simulink model "reaction_pendulum"  (R2021b)
settings: Solver=FixedStepDiscrete  StartTime=0.0  StopTime=20  FixedStep=h  RelTol=1e-3  EnableMultiTasking=on
PreLoadFcn:
  | warning('off','MATLAB:dispatcher:InexactMatch');
InitFcn:
  | hwinit
undefined symbols (not defined in the file or in its folder): estimate_A, estimate_C, estimate_D
libraries: slident x2, dspsrcs4 x1
settings Model: SimulationMode=external  ExtModeTrigDuration=100000  Creator=user  LastModifiedBy=nstienen
settings SolverCC: AlgebraicLoopSolver=TrustRegion
settings DataIOCC: SaveFormat=Array  SignalLoggingSaveFormat=ModelDataLogs  SaveOutput=off  SignalLogging=off  DSMLogging=off  SaveTime=off  ReturnWorkspaceOutputs=off
settings OptimizationCC: ExpressionDepthLimit=2147483647  LifeSpan=inf
settings DebuggingCC: UnderspecifiedInitializationDetection=Classic  MergeDetectMultiDrivingBlocksExec=none  SolverPrmCheckMsg=warning  FcnCallInpInsideContextMsg=warning  StateNameClashWarn=warning  SFUnexpectedBacktrackingDiag=warning  SFNoUnconditionalDefaultTransitionDiag=warning  SFExecutionAtInitializationDiag=none  SFMachineParentedDataDiag=warning  ArithmeticOperatorsInVariantConditions=warning
settings HardwareCC: ProdBitPerPointer=32  ProdBitPerSizeT=32  ProdBitPerPtrDiffT=32  ProdLargestAtomicFloat=None  ProdIntDivRoundTo=Undefined  ProdEndianess=Unspecified  ProdWordSize=32  ProdHWDeviceType=32-bit Generic
settings ModelReferenceCC: PropagateSignalLabelsOutOfModel=off
settings SFSimCC: SimUseLocalCustomCode=off  CustomCodeUndefinedFunction=UseInterfaceOnly
settings RTWCC: Description=rpend RTDAC/USB2 (Visual C/C++)  SystemTargetFile=rtcon_rpend_usb2.tlc  TemplateMakefile=rtcon_rpend_vc_usb2_x64.tmf  RTWUseLocalCustomCode=off
settings CodeAppCC: StateflowObjectComments=on
settings STFCustomTargetCC: ModelReferenceCompliant=off  CombineOutputUpdateFcns=on  MatFileLogging=on  GRTInterface=off  SystemTargetFile=rtcon_rpend_usb2.tlc
settings GRTTargetCC: TargetLangStandard=C89/C90 (ANSI)  ModelReferenceCompliant=off  ParMdlRefBuildCompliant=off  CompOptLevelCompliant=off  ConcurrentExecutionCompliant=off  CPPClassGenCompliant=off  UseToolchainInfoCompliant=off  ExtMode=on  ExtModeMexFile=rtcon_ext_comm
settings ConfigComp: CovMetricSettings=dw  CovSaveCumulativeToWorkspaceVar=on  CovSaveSingleToWorkspaceVar=on  CovExternalEMLEnable=off  CovSFcnEnable=off

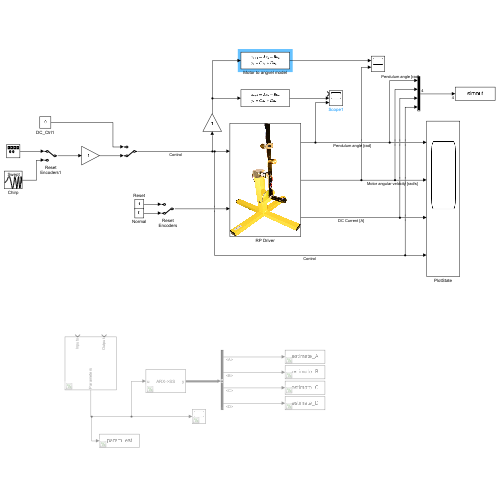
[thumbnail: Simulink's stored preview of the top-level diagram]
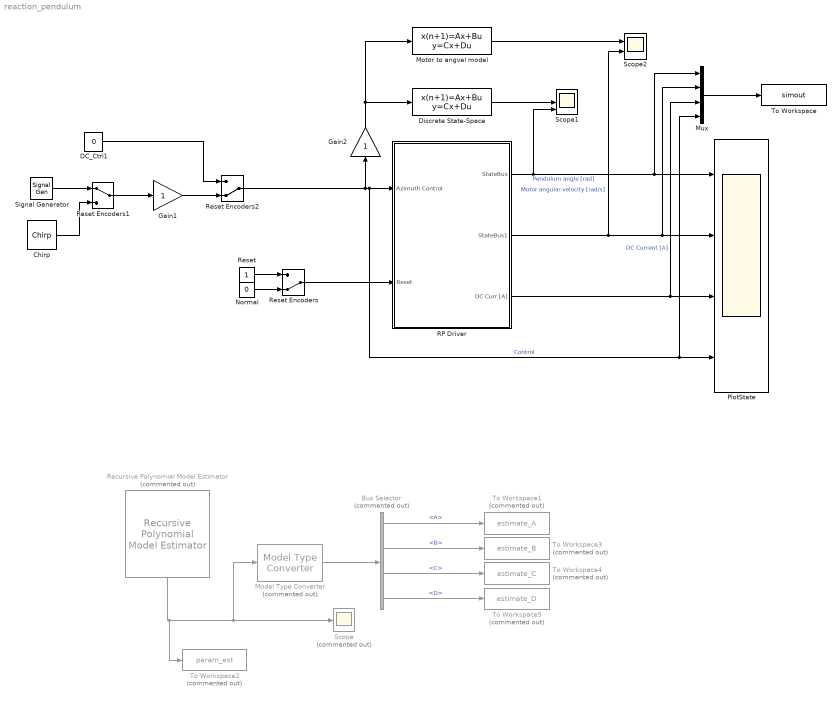
== system reaction_pendulum ==
  Bus Selector : BusSelector  Commented=on  OutputSignals=A,B,C,D
  Chirp : dspsrcs4/Chirp  sweep=Swept cosine  mode=Unidirectional  f0=0.1  f1=0.8  t1=30  Tsweep=30  phase=0  Ts=0.05  spf=1  datatype=Double  OutputFrames=off
  DC_Ctrl1 : Constant  Value=0
  Discrete State-Space : DiscreteStateSpace  A=estimate_A  B=estimate_B.'  C=estimate_C  D=estimate_D  SampleTime=-1
  Gain1 : Gain
  Gain2 : Gain
  Model Type Converter : slident/Estimators/Model Type Converter  Commented=on  InputModelType=ARX
      settings: SourceProductBaseCode=ID
  Motor to angvel model : DiscreteStateSpace  A=0.9683  B=19.81  D=0  SampleTime=-1
  Mux : Mux
  Normal : Constant  Value=0
  PlotState : Scope  NumInputPorts=4
  RP Driver : Subsystem
      mask Display: image(imread('rwp.JPG'))
  Recursive Polynomial Model Estimator : slident/Estimators/Recursive Polynomial Model Estimator  Commented=on  ModelStructure=ARX  InitialEstimateSource=None  A0=3  B0=1  C0=1  D0=1  F0=2  nk=1  P0=1e4  InitialInputs=0  InitialOutputs=0  History=Infinite  WindowLength=200  EstimationMethod=Kalman Filter  AdaptationParameter=1  HasTimeVaryingAdaptationParameter=off  NormalizationBias=eps  OutputError=off  OutputP=off  AddEnablePort=off  InputProcessing=Sample-based  Ts=-1
      settings: SourceProductBaseCode=ID
  Reset : Constant
  Reset Encoders : ManualSwitch  CurrentSetting=0
  Reset Encoders1 : ManualSwitch
  Reset Encoders2 : ManualSwitch  CurrentSetting=0
  Scope : Scope  Commented=on
  Scope1 : Scope  NumInputPorts=3
  Scope2 : Scope  NumInputPorts=2
  Signal Generator : SignalGenerator  Frequency=1/2
  To Workspace : ToWorkspace  VariableName=simout  SaveFormat=Structure With Time  SampleTime=-1
      settings: Save2DSignal=2-D array (concatenate along first dimension)
  To Workspace1 : ToWorkspace  Commented=on  VariableName=estimate_A  SampleTime=-1
      settings: MaxDataPoints=1
  To Workspace2 : ToWorkspace  Commented=on  VariableName=param_est  SaveFormat=Structure With Time  SampleTime=-1
  To Workspace3 : ToWorkspace  Commented=on  VariableName=estimate_B  SampleTime=-1
      settings: MaxDataPoints=1
  To Workspace4 : ToWorkspace  Commented=on  VariableName=estimate_C  SampleTime=-1
      settings: MaxDataPoints=1
  To Workspace5 : ToWorkspace  Commented=on  VariableName=estimate_D  SampleTime=-1
      settings: MaxDataPoints=1
  wires:
  Normal/1 -> Reset Encoders/2
  Reset/1 -> Reset Encoders/1
  Reset Encoders/1 -> RP Driver/2(Reset)
  RP Driver/3(DC Curr [A]) -> Mux/3, PlotState/3  "DC Current [A]"
  Reset Encoders2/1 -> Gain2/1, Mux/4, PlotState/4, RP Driver/1(Azimuth Control)  "Control"
  DC_Ctrl1/1 -> Reset Encoders2/1
  RP Driver/2(StateBus1) -> Scope2/2, Mux/2, PlotState/2  "Motor angular velocity [rad/s]"
  Gain1/1 -> Reset Encoders2/2
  RP Driver/1(StateBus) -> Scope1/3, Mux/1, PlotState/1  "Pendulum angle [rad]"
  Mux/1 -> To Workspace/1
  Reset Encoders1/1 -> Gain1/1
  Signal Generator/1 -> Reset Encoders1/1
  Chirp/1 -> Reset Encoders1/2
  Recursive Polynomial Model Estimator/1 -> To Workspace2/1, Model Type Converter/1, Scope/1
  Model Type Converter/1 -> Bus Selector/1
  Bus Selector/1 -> To Workspace1/1  "<A>"
  Bus Selector/3 -> To Workspace4/1  "<C>"
  Bus Selector/4 -> To Workspace5/1  "<D>"
  Bus Selector/2 -> To Workspace3/1  "<B>"
  Discrete State-Space/1 -> Scope1/2
  Gain2/1 -> Motor to angvel model/1, Discrete State-Space/1
  Motor to angvel model/1 -> Scope2/1

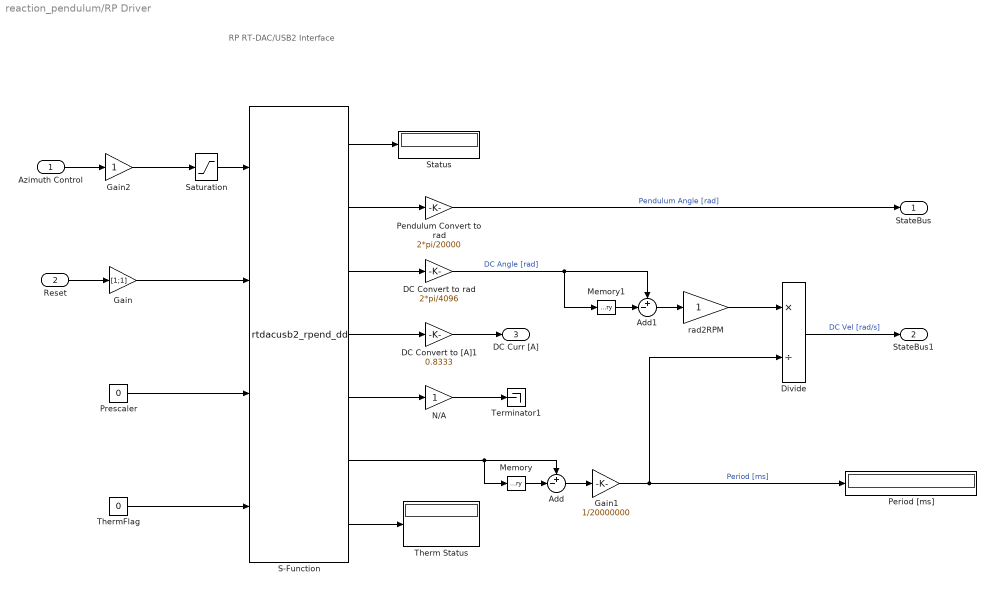
== system reaction_pendulum/RP Driver ==
  note: RP RT-DAC/USB2
      | Interface
  Azimuth Control : Inport
  Reset : Inport  Port=2
  Add : Sum  Inputs=+-|
  Add1 : Sum  Inputs=+-|
  DC Convert to [A]1 : Gain  Gain=0.8333  SaturateOnIntegerOverflow=on  OutDataTypeStr=Inherit: Same as input  ParamDataTypeStr=Inherit: Same as input
  DC Convert to rad : Gain  Gain=2*pi/4096  SaturateOnIntegerOverflow=on  OutDataTypeStr=Inherit: Same as input  ParamDataTypeStr=Inherit: Same as input
  Divide : Product  Inputs=*/
  Gain : Gain  Gain=[1;1]
  Gain1 : Gain  Gain=1/20000000
  Gain2 : Gain
  Memory : Memory
  Memory1 : Memory
  N/A : Gain  SaturateOnIntegerOverflow=on  OutDataTypeStr=Inherit: Same as input  ParamDataTypeStr=Inherit: Same as input
  Pendulum Convert to rad : Gain  Gain=2*pi/20000  SaturateOnIntegerOverflow=on  OutDataTypeStr=Inherit: Same as input  ParamDataTypeStr=Inherit: Same as input
  Period [ms] : Display
  Prescaler : Constant  Value=0
  S-Function : S-Function  FunctionName=rtdacusb2_rpend_dd  Parameters=1, h  SFunctionDeploymentMode=off  EnableBusSupport=off
  Saturation : Saturate  UpperLimit=1  LowerLimit=-1
  Status : Display
  Terminator1 : Terminator
  Therm Status : Display
  ThermFlag : Constant  Value=0
  rad2RPM : Gain  SaturateOnIntegerOverflow=on  OutDataTypeStr=Inherit: Same as input  ParamDataTypeStr=Inherit: Same as input
  StateBus : Outport  VectorParamsAs1DForOutWhenUnconnected=off
  StateBus1 : Outport  Port=2  VectorParamsAs1DForOutWhenUnconnected=off
  DC Curr [A] : Outport  Port=3  VectorParamsAs1DForOutWhenUnconnected=off
  wires:
  S-Function/7 -> Therm Status/1
  S-Function/5 -> N/A/1
  S-Function/4 -> DC Convert to [A]1/1
  ThermFlag/1 -> S-Function/4
  Prescaler/1 -> S-Function/3
  Gain/1 -> S-Function/2
  DC Convert to [A]1/1 -> DC Curr [A]/1
  Divide/1 -> StateBus1/1  "DC Vel [rad/s]"
  rad2RPM/1 -> Divide/1
  Add1/1 -> rad2RPM/1
  Memory1/1 -> Add1/2
  N/A/1 -> Terminator1/1
  S-Function/6 -> Add/1, Memory/1
  Gain2/1 -> Saturation/1
  Gain1/1 -> Period [ms]/1, Divide/2  "Period [ms]"
  Add/1 -> Gain1/1
  Memory/1 -> Add/2
  DC Convert to rad/1 -> Add1/1, Memory1/1  "DC Angle [rad]"
  S-Function/3 -> DC Convert to rad/1
  Pendulum Convert to rad/1 -> StateBus/1  "Pendulum Angle [rad]"
  S-Function/2 -> Pendulum Convert to rad/1
  S-Function/1 -> Status/1
  Saturation/1 -> S-Function/1
  Reset/1 -> Gain/1
  Azimuth Control/1 -> Gain2/1
